simulink model "Prak1Aufg3Simulink"  (Simulink 7.7)
settings: Solver=ode3  StartTime=0.0  StopTime=120  FixedStep=0.002  RelTol=1e-3
settings Model: Creator=Milena  LastModifiedBy=hexren

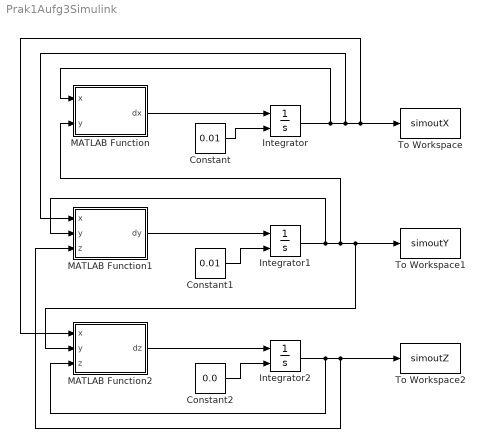
== system Prak1Aufg3Simulink ==
  Constant : Constant  Value=0.01
  Constant1 : Constant  Value=0.01
  Constant2 : Constant  Value=0.0
  Integrator : Integrator  InitialConditionSource=external
  Integrator1 : Integrator  InitialConditionSource=external
  Integrator2 : Integrator  InitialConditionSource=external
  MATLAB Function : Stateflow chart  TreatAsAtomicUnit=on
  MATLAB Function1 : Stateflow chart  TreatAsAtomicUnit=on
  MATLAB Function2 : Stateflow chart  TreatAsAtomicUnit=on
  To Workspace : ToWorkspace  VariableName=simoutX  SampleTime=-1  SaveFormat=Array
  To Workspace1 : ToWorkspace  VariableName=simoutY  SampleTime=-1  SaveFormat=Array
  To Workspace2 : ToWorkspace  VariableName=simoutZ  SampleTime=-1  SaveFormat=Array
  wires:
  MATLAB Function/1(dx) -> Integrator/1
  MATLAB Function1/1(dy) -> Integrator1/1
  MATLAB Function2/1(dz) -> Integrator2/1
  Constant/1 -> Integrator/2
  Constant1/1 -> Integrator1/2
  Constant2/1 -> Integrator2/2
  Integrator/1 -> MATLAB Function/1(x), To Workspace/1, MATLAB Function2/1(x), MATLAB Function1/1(x)
  Integrator1/1 -> MATLAB Function1/2(y), MATLAB Function/2(y), To Workspace1/1, MATLAB Function2/2(y)
  Integrator2/1 -> MATLAB Function2/3(z), To Workspace2/1, MATLAB Function1/3(z)

== matlab function MATLAB Function1 ==
  data: x input double; y input double; z input double; dy output double
function dy = dglY(x, y, z)
%#codegen

dy = (40 - z) * x - y;

== matlab function MATLAB Function ==
  data: x input double; y input double; dx output double
function dx = dglX(x, y)
%#codegen

dx = -10 * (x - y);

== matlab function MATLAB Function2 ==
  data: x input double; y input double; z input double; dz output double
function dz = dglZ(x, y, z)
%#codegen

dz = x * y -2.67 * z;
